simulink model "coolant_flow_example"  (R2023a)
settings: Solver=VariableStepAuto  StartTime=0.0  StopTime=10.0  RelTol=1e-3
libraries: component_lib x7
settings Model: Creator=maxjo  LastModifiedBy=maxjo

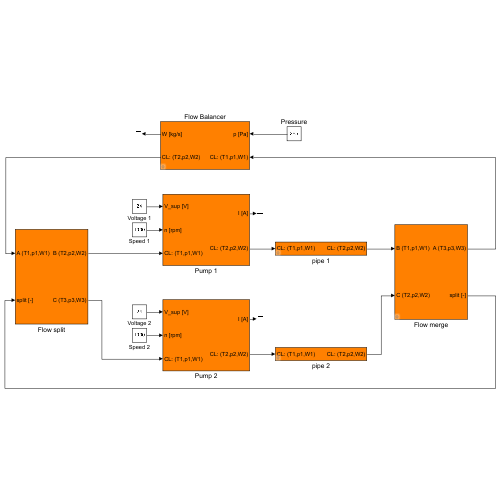
[thumbnail: Simulink's stored preview of the top-level diagram]
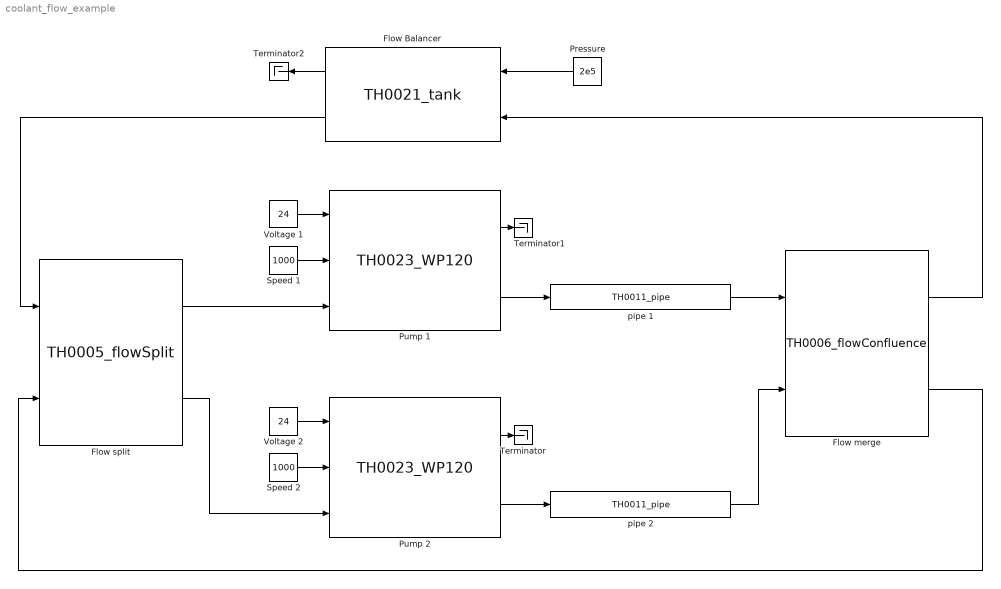
== system coolant_flow_example ==
  Flow Balancer : component_lib/Thermal Systems/TH0021_tank  V=5e-3  T0=273.15 + 80
  Flow merge : component_lib/Thermal Systems/TH0006_flowConfluence  gain=0.01
  Flow split : component_lib/Thermal Systems/TH0005_flowSplit  SystemSampleTime=-1  VariantActivationTime=update diagram  Latency=0  AutoFrameSizeCalculation=off
  Pressure : Constant  Value=2e5
  Pump 1 : component_lib/Thermal Systems/TH0023_WP120  SystemSampleTime=-1  VariantActivationTime=update diagram  Latency=0  AutoFrameSizeCalculation=off
  Pump 2 : component_lib/Thermal Systems/TH0023_WP120  SystemSampleTime=-1  VariantActivationTime=update diagram  Latency=0  AutoFrameSizeCalculation=off
  Speed 1 : Constant  Value=1000
  Speed 2 : Constant  Value=1000
  Terminator : Terminator
  Terminator1 : Terminator
  Terminator2 : Terminator
  Voltage 1 : Constant  Value=24
  Voltage 2 : Constant  Value=24
  pipe 1 : component_lib/Thermal Systems/TH0011_pipe  d=5e-2  L=1  e=0.006e-3  T_0=273 + 20
  pipe 2 : component_lib/Thermal Systems/TH0011_pipe  d=5e-2  L=1  e=0.006e-3  T_0=273 + 20
  wires:
  Voltage 1/1 -> Pump 1/1
  Speed 1/1 -> Pump 1/2
  Voltage 2/1 -> Pump 2/1
  Speed 2/1 -> Pump 2/2
  Pump 2/1 -> Terminator/1
  Pump 1/1 -> Terminator1/1
  Flow split/1 -> Pump 1/3
  Flow split/2 -> Pump 2/3
  Pump 1/2 -> pipe 1/1
  pipe 1/1 -> Flow merge/1
  Pump 2/2 -> pipe 2/1
  pipe 2/1 -> Flow merge/2
  Flow merge/2 -> Flow split/2
  Flow Balancer/1 -> Terminator2/1
  Flow merge/1 -> Flow Balancer/2
  Flow Balancer/2 -> Flow split/1
  Pressure/1 -> Flow Balancer/1
